simulink model "HILClimbers_Integrated_V5"  (R2021a)
settings: Solver=VariableStepAuto  StartTime=0.0  StopTime=10.0  RelTol=1e-3
undefined symbols (not defined in the file): brake
settings Model: OrderedModelArguments=off  Creator=Sai229  LastModifiedBy=Sai229

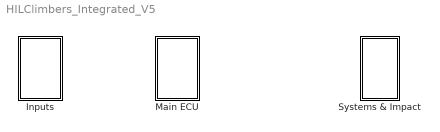
== system HILClimbers_Integrated_V5 ==
  Inputs : Subsystem
  Main ECU : Subsystem
  Systems & Impact : Subsystem

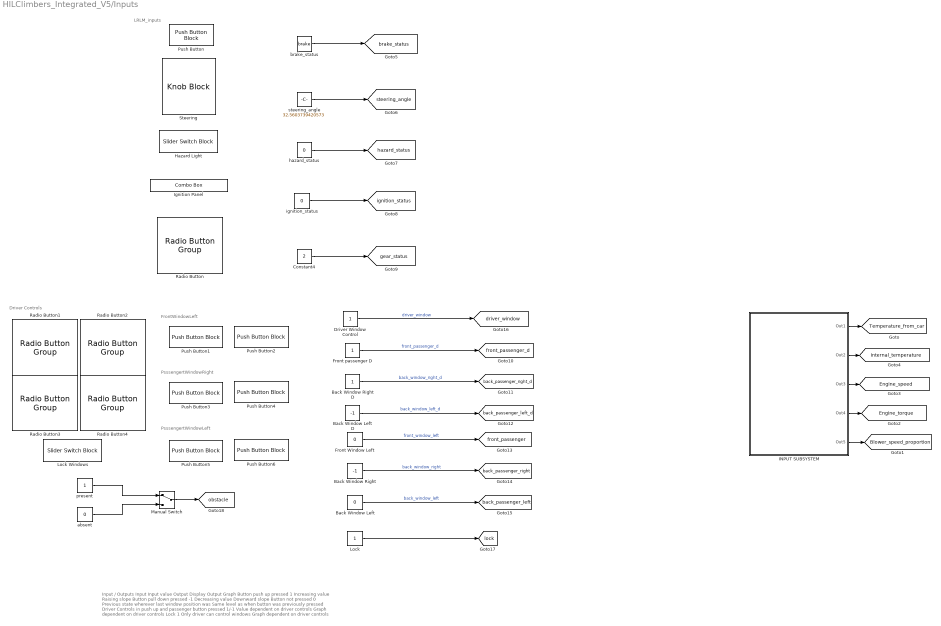
== system HILClimbers_Integrated_V5/Inputs ==
  note: LRLM_inputs
  note: Input / Outputs
      |
      | Input
      | Input value
      | Output Display
      | Output Graph
      |
      | Button push up pressed
      | 1
      | Increasing value
      | Raising slope
      |
      | Button pull down pressed
      | -1
      | Decreasing value
      | Downward slope
      |
      | Button not pressed
      | 0
      | Previous state wherever last window position was
      | Same level as when button was previously pressed
      |
      | Driver Controls in push up and passenger button pressed
      | 1/-1
      | Value dependent on driver controls
      | Graph dependent on driver controls
      |
      | Lock
      | 1
      | Only driver can control windows
      | Graph dependent on driver controls
  note: FrontWindowLeft
  note: Driver Controls
  note: PsssengertWindowRight
  note: PsssengertWindowLeft
  Back Window Left : Constant  Value=0
  Back Window Left D : Constant  Value=-1
  Back Window Right : Constant  Value=-1
  Back Window Right D : Constant
  Constant4 : Constant  Value=2
  Driver Window Control : Constant
  Front Window Left : Constant  Value=0
  Front passenger D : Constant
  Hazard Light : SliderSwitchBlock  LabelPosition=Hide
      settings: Values={{'Off', 'On'}, [0 1]}
  INPUT SUBSYSTEM : Subsystem
  Ignition Panel : ComboBox  LabelPosition=Hide  SelectedLabel=Key Not Inserted
      settings: Values={{'Key Not Inserted', 'Key Inserted', 'Pre-Ignition', 'Vehicle Started'}, [0 1 2 3]}
  Lock : Constant
  Lock Windows : SliderSwitchBlock
      settings: Values={{'Unlock', 'Lock'}, [0 1]}
  Manual Switch : ManualSwitch
  Push Button : PushButtonBlock  ButtonText=Brake
  Push Button1 : PushButtonBlock  ButtonText=Push up window
  Push Button2 : PushButtonBlock  ButtonText=Pull down window  OnValue=-1
  Push Button3 : PushButtonBlock  ButtonText=Push up window
  Push Button4 : PushButtonBlock  ButtonText=Pull down window  OnValue=-1
  Push Button5 : PushButtonBlock  ButtonText=Push up window
  Push Button6 : PushButtonBlock  ButtonText=Pull down window  OnValue=-1
  Radio Button : RadioButtonGroup  LabelPosition=Hide  SelectedLabel=Park  ButtonGroupName=Gear
      settings: Values={{'Neutral', 'Drive', 'Park', 'Reverse'}, [0 1 2 3]}
  Radio Button1 : RadioButtonGroup  LabelPosition=Hide  SelectedLabel=Open  ButtonGroupName=Driver Window Controls
      settings: Values={{'Open', 'Stop', 'Close'}, [1 0 -1]}
  Radio Button2 : RadioButtonGroup  LabelPosition=Hide  SelectedLabel=Open  ButtonGroupName=Front Passenger
      settings: Values={{'Open', 'Stop', 'Close'}, [1 0 -1]}
  Radio Button3 : RadioButtonGroup  LabelPosition=Hide  SelectedLabel=Open  ButtonGroupName=Back Window Right
      settings: Values={{'Open', 'Stop', 'Close'}, [1 0 -1]}
  Radio Button4 : RadioButtonGroup  LabelPosition=Hide  SelectedLabel=Close  ButtonGroupName=Back Window Left
      settings: Values={{'Open', 'Stop', 'Close'}, [1 0 -1]}
  Steering : KnobBlock  LabelPosition=Hide  ScaleMin=-50  ScaleMax=50  TickInterval=10
  absent : Constant  Value=0
  brake_status : Constant  Value=brake
  hazard_status : Constant  Value=0
  ignition_status : Constant  Value=0
  present : Constant
  steering_angle : Constant  Value=32.5603739420573
  tag scope: Blower_speed_proportion=global, Engine_speed=global, Engine_torque=global, Internal_temperature=global, Temperature_from_car=global, back_passenger_left=global, back_passenger_left_d=global, back_passenger_right=global, back_passenger_right_d=global, brake_status=global, driver_window=global, front_passenger=global, front_passenger_d=global, gear_status=global, hazard_status=global, ignition_status=global, lock=global, obstacle=global, steering_angle=global
  wires:
  steering_angle/1 -> [steering_angle]
  INPUT SUBSYSTEM/2(Out2) -> [Internal_temperature]
  INPUT SUBSYSTEM/4(Out4) -> [Engine_torque]
  present/1 -> Manual Switch/1
  ignition_status/1 -> [ignition_status]
  INPUT SUBSYSTEM/1(Out1) -> [Temperature_from_car]
  INPUT SUBSYSTEM/3(Out3) -> [Engine_speed]
  INPUT SUBSYSTEM/5(Out5) -> [Blower_speed_proportion]
  Constant4/1 -> [gear_status]
  hazard_status/1 -> [hazard_status]
  brake_status/1 -> [brake_status]
  Front Window Left/1 -> [front_passenger]  "front_window_left"
  Driver Window Control/1 -> [driver_window]  "driver_window"
  absent/1 -> Manual Switch/2
  Back Window Right D/1 -> [back_passenger_right_d]  "back_window_right_d"
  Back Window Left D/1 -> [back_passenger_left_d]  "back_window_left_d"
  Front passenger D/1 -> [front_passenger_d]  "front_passenger_d"
  Back Window Right/1 -> [back_passenger_right]  "back_window_right"
  Back Window Left/1 -> [back_passenger_left]  "back_window_left"
  Lock/1 -> [lock]
  Manual Switch/1 -> [obstacle]

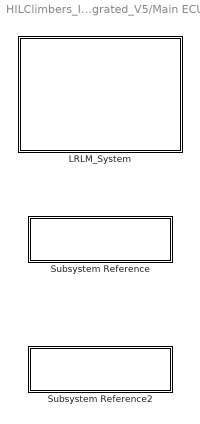
== system HILClimbers_Integrated_V5/Main ECU ==
  LRLM_System : Subsystem  ReferencedSubsystem=LRLM_ECU  time_period=1
  Subsystem Reference : Subsystem  ReferencedSubsystem=Power_Window_ECU
  Subsystem Reference2 : Subsystem  ReferencedSubsystem=HVAC_ECU

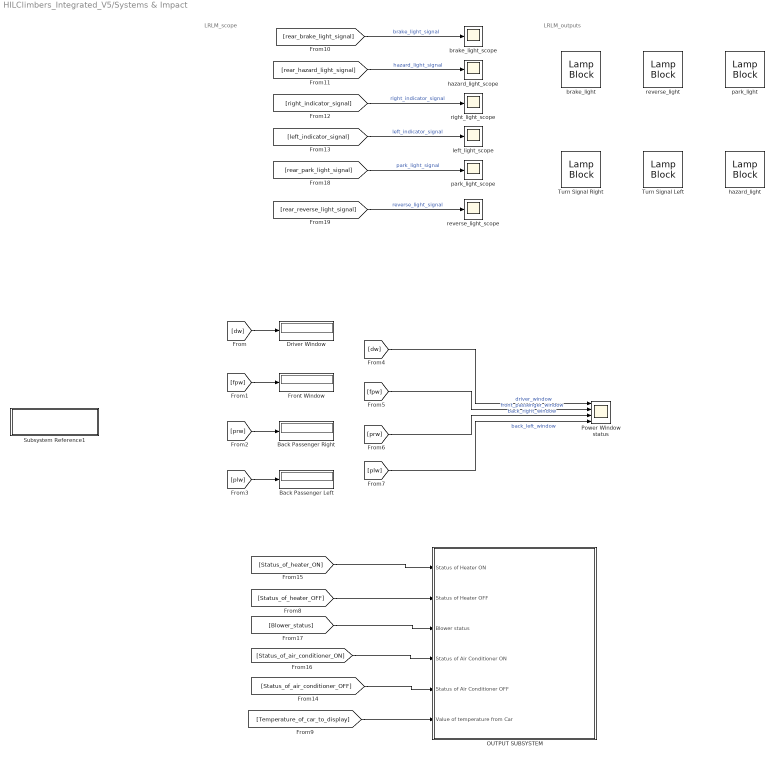
== system HILClimbers_Integrated_V5/Systems & Impact ==
  note: LRLM_outputs
  note: LRLM_scope
  Back Passenger Left : Display
  Back Passenger Right : Display
  Driver Window : Display
  Front Window : Display
  OUTPUT SUBSYSTEM : Subsystem
  Power Window status : Scope  NumInputPorts=4
  Subsystem Reference1 : Subsystem  ReferencedSubsystem=Power_Window_System_and_Impact
  Turn Signal Left : LampBlock  LabelPosition=Hide  Icon=TurnSignalLeft
  Turn Signal Right : LampBlock  LabelPosition=Hide  Icon=TurnSignalRight
  brake_light : LampBlock  LabelPosition=Hide  Icon=LightingSwitch
  brake_light_scope : Scope
  hazard_light : LampBlock  LabelPosition=Hide  Icon=Hazards
  hazard_light_scope : Scope
  left_light_scope : Scope
  park_light : LampBlock  Icon=ParkingAssistance
  park_light_scope : Scope
  reverse_light : LampBlock  Icon=RearFogLight
  reverse_light_scope : Scope
  right_light_scope : Scope
  wires:
  [Status_of_air_conditioner_OFF] -> OUTPUT SUBSYSTEM/5(Status of Air Conditioner OFF)
  [Temperature_of_car_to_display] -> OUTPUT SUBSYSTEM/6(Value of temperature from Car)
  [Status_of_air_conditioner_ON] -> OUTPUT SUBSYSTEM/4(Status of Air Conditioner ON)
  [Blower_status] -> OUTPUT SUBSYSTEM/3(Blower status)
  [Status_of_heater_OFF] -> OUTPUT SUBSYSTEM/2(Status of Heater OFF)
  [prw] -> Back Passenger Right/1
  [dw] -> Driver Window/1
  [plw] -> Power Window status/4  "back_left_window"
  [fpw] -> Front Window/1
  [fpw] -> Power Window status/2  "front_passenger_window"
  [prw] -> Power Window status/3  "back_right_window"
  [dw] -> Power Window status/1  "driver_window"
  [plw] -> Back Passenger Left/1
  [Status_of_heater_ON] -> OUTPUT SUBSYSTEM/1(Status of Heater ON)
  [right_indicator_signal] -> right_light_scope/1  "right_indicator_signal"
  [left_indicator_signal] -> left_light_scope/1  "left_indicator_signal"
  [rear_park_light_signal] -> park_light_scope/1  "park_light_signal"
  [rear_brake_light_signal] -> brake_light_scope/1  "brake_light_signal"
  [rear_hazard_light_signal] -> hazard_light_scope/1  "hazard_light_signal"
  [rear_reverse_light_signal] -> reverse_light_scope/1  "reverse_light_signal"

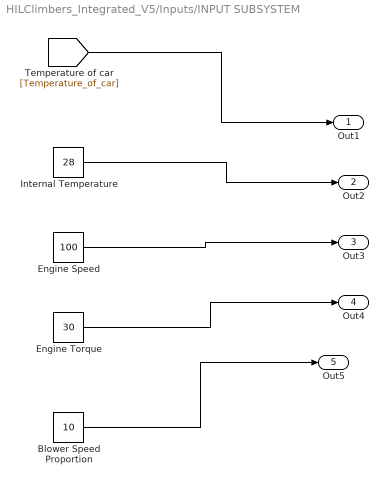
== system HILClimbers_Integrated_V5/Inputs/INPUT SUBSYSTEM ==
  Blower Speed Proportion : Constant  Value=10
  Engine Speed : Constant  Value=100
  Engine Torque : Constant  Value=30
  Internal Temperature : Constant  Value=28
  Out1 : Outport
  Out2 : Outport  Port=2
  Out3 : Outport  Port=3
  Out4 : Outport  Port=4
  Out5 : Outport  Port=5
  wires:
  Engine Speed/1 -> Out3/1
  Blower Speed Proportion/1 -> Out5/1
  Internal Temperature/1 -> Out2/1
  Engine Torque/1 -> Out4/1
  [Temperature_of_car] -> Out1/1

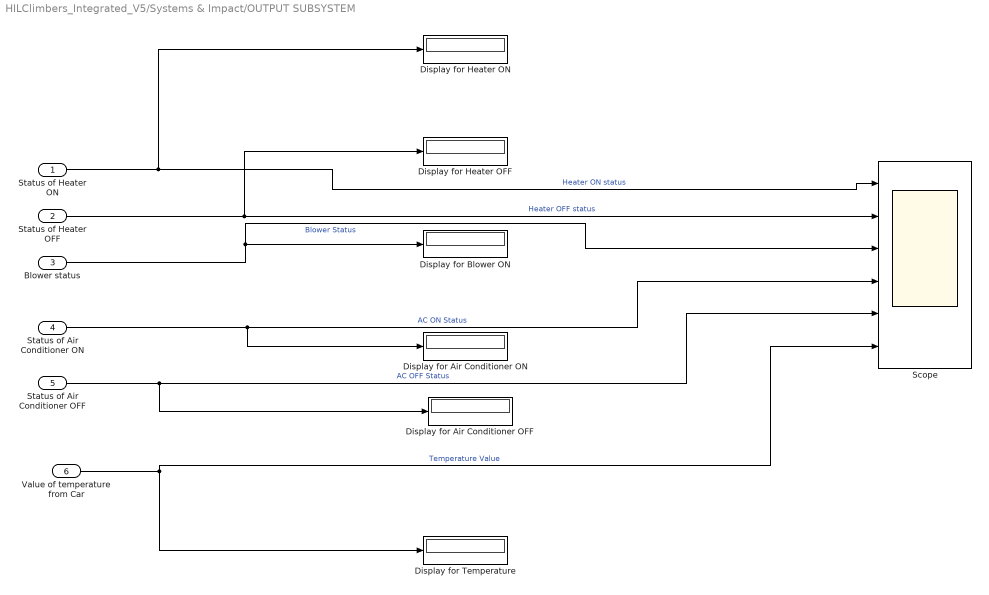
== system HILClimbers_Integrated_V5/Systems & Impact/OUTPUT SUBSYSTEM ==
  Status of Heater ON : Inport
  Status of Heater OFF : Inport  Port=2
  Blower status : Inport  Port=3
  Status of Air Conditioner ON : Inport  Port=4
  Status of Air Conditioner OFF : Inport  Port=5
  Value of temperature from Car : Inport  Port=6
  Display for Air Conditioner OFF : Display
  Display for Air Conditioner ON : Display
  Display for Blower ON : Display
  Display for Heater OFF : Display
  Display for Heater ON : Display
  Display for Temperature : Display
  Scope : Scope  NumInputPorts=6
  wires:
  Status of Air Conditioner ON/1 -> Scope/4, Display for Air Conditioner ON/1  "AC ON Status"
  Blower status/1 -> Scope/3, Display for Blower ON/1  "Blower Status"
  Status of Heater ON/1 -> Scope/1, Display for Heater ON/1  "Heater ON status"
  Value of temperature from Car/1 -> Scope/6, Display for Temperature/1  "Temperature Value"
  Status of Heater OFF/1 -> Scope/2, Display for Heater OFF/1  "Heater OFF status"
  Status of Air Conditioner OFF/1 -> Scope/5, Display for Air Conditioner OFF/1  "AC OFF Status"
